simulink model "Simulink_EbolaControlSISO"  (R2021b)
settings: Solver=VariableStepAuto  StartTime=0.0  StopTime=1000.0  FixedStep=0.00126939799450362  RelTol=1e-3
model workspace (MAT data in the model file):
  Beta = 1.89e-07
  C = 8
  Delta = 0.0055
  P = 378
  U = 500
  Uu = 250
  V0 = 1.05
  u = 250
undefined symbols (not defined in the file or in its folder): sigbuilder_block
settings Model: Creator=Camilo  LastModifiedBy=Camilo
settings DataIOCC: SaveFormat=Array  OutputTimes=tout

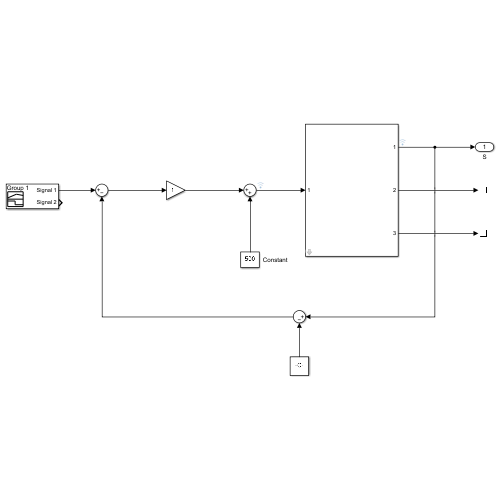
[thumbnail: Simulink's stored preview of the top-level diagram]
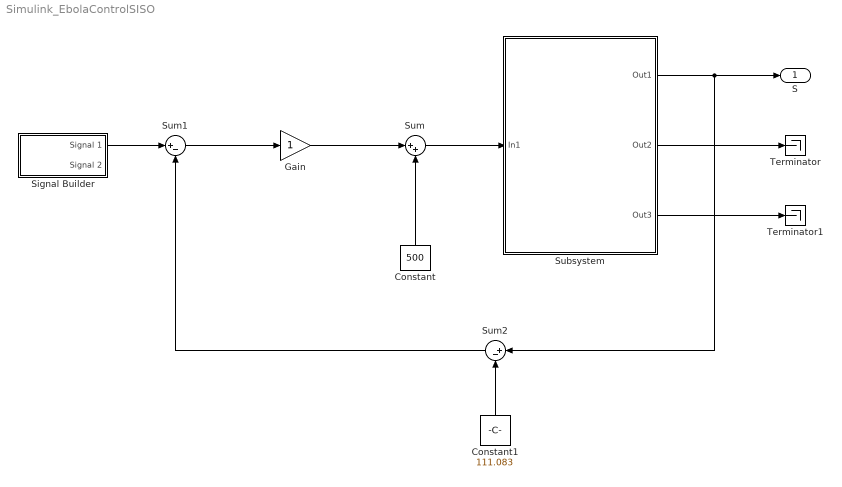
== system Simulink_EbolaControlSISO ==
  Constant : Constant  Value=500  VectorParams1D=off  SampleTime=-1
  Constant1 : Constant  Value=111.083
  Gain : Gain
  Signal Builder : Subsystem  Tag=STV Subsys  LoadFcn=sigbuilder_block('load',[429.6 149.4 550.8 400.2 ]);  StartFcn=sigbuilder_block('start');  StopFcn=sigbuilder_block('stop');  ClipboardFcn=sigbuilder_block('clipboard');  mask(Sigbuilder block){tuvar=[0:10]}
      mask help: Simulink:masks:SigbuilderBlock_MD
      mask init:
      | if ~strcmp(get_param(bdroot(gcbh),'SimulationStatus'),'stopped') tuvar = sigbuilder_block('maskInit'); end
      settings: CopyFcn=sigbuilder_block('copy');  DeleteFcn=sigbuilder_block('delete');  ModelCloseFcn=sigbuilder_block('modelClose');  PreSaveFcn=sigbuilder_block('preSave');  PauseFcn=sigbuilder_block('pause');  ContinueFcn=sigbuilder_block('continue');  NameChangeFcn=sigbuilder_block('namechange');  OpenFcn=sigbuilder_block('open',[429.6 149.4 550.8 400.2 ]);  CloseFcn=sigbuilder_block('close');
      mask Display: plot(0, 0, 100, 100,[2, 2, 32, 32, 2], [68, 8, 8, 68, 68],[32, 2], [38, 38], [32, 19, 2],[53, 60, 44], [32, 17, 17, 2],[16, 16, 31, 31]);txt = getActiveGroup(gcbh);text(2, 100, txt,'verticalAlignment', 'top');
  Subsystem : Subsystem  mask{V0=23560849.185935, Delta=1e-3, P=378, C=8.02, Beta=1.91e-7}
  Sum : Sum  Inputs=|++
  Sum1 : Sum  Inputs=|+-
  Sum2 : Sum  Inputs=|+-
  Terminator : Terminator
  Terminator1 : Terminator
  S : Outport
  wires:
  Subsystem/1(Out1) -> Sum2/1, S/1
  Subsystem/2(Out2) -> Terminator/1
  Subsystem/3(Out3) -> Terminator1/1
  Sum/1 -> Subsystem/1(In1)
  Constant/1 -> Sum/2
  Gain/1 -> Sum/1
  Sum1/1 -> Gain/1
  Constant1/1 -> Sum2/2
  Sum2/1 -> Sum1/2
  Signal Builder/1(Signal 1) -> Sum1/1

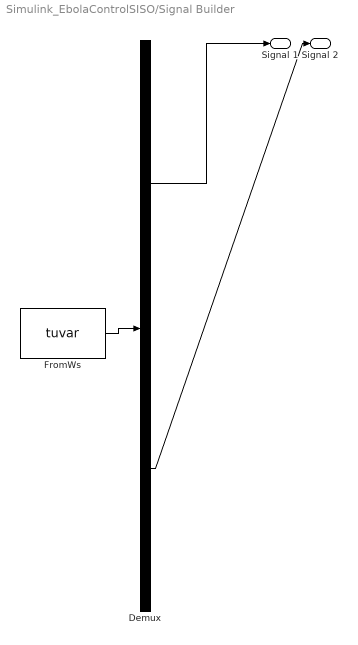
== system Simulink_EbolaControlSISO/Signal Builder ==
  Demux : Demux  Tag=STV Demux  Outputs=2
      settings: DisplayOption=none
  FromWs : FromWorkspace  Tag=STV FromWs  VariableName=tuvar
      SigBuilderData=|
      | common.afterFinalStr = 'Extrapolate'
      | common.sampleTime = 0
      | dataSet.timeRange = [0 10]
      | dataSet.name = 'Group 1'
      | sbobj.Groups.Name = 'Group 1'
      | sbobj.Groups.Signals(1).Name = 'Signal 1'
      | sbobj.Groups.Signals(1).XData = [0 10]
      | sbobj.Groups.Signals(1).YData = [0 0]
      | sbobj.Groups.Signals(2).Name = 'Signal 2'
      | sbobj.Groups.Signals(2).XData = [0 4 4 6 6 10]
      | sbobj.Groups.Signals(2).YData = [0 0 1 1 0 0]
  Signal 1 : Outport  Tag=STV Outport
  Signal 2 : Outport  Tag=STV Outport  Port=2
  wires:
  Demux/1 -> Signal 1/1
  FromWs/1 -> Demux/1
  Demux/2 -> Signal 2/1

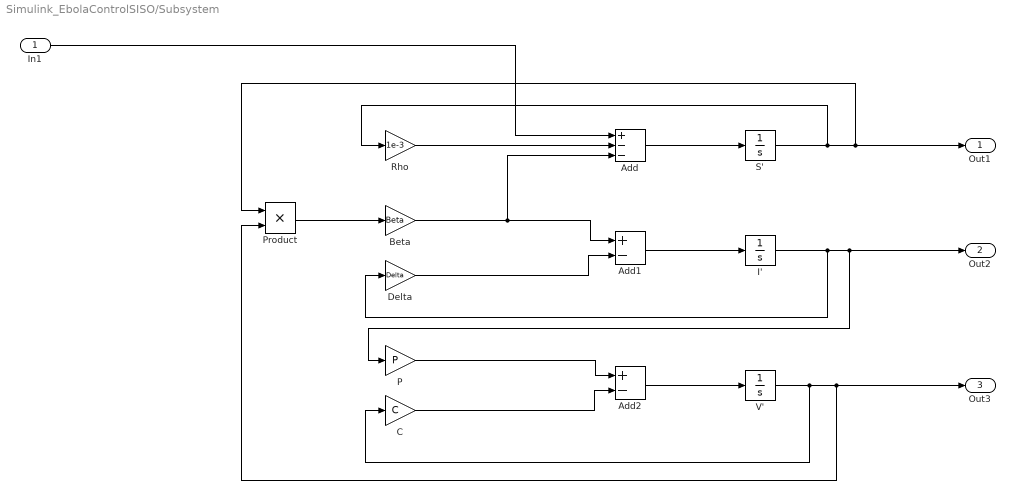
== system Simulink_EbolaControlSISO/Subsystem ==
  In1 : Inport
  Add : Sum  Inputs=+--
  Add1 : Sum  Inputs=+-
  Add2 : Sum  Inputs=+-
  Beta : Gain  Gain=Beta
  C : Gain  Gain=C
  Delta : Gain  Gain=Delta
  I' : Integrator  InitialCondition=4.99988917e+05  LimitOutput=on  LowerSaturationLimit=0
  P : Gain  Gain=P
  Product : Product
  Rho : Gain  Gain=1e-3
  S' : Integrator  InitialCondition=111.083  LimitOutput=on  LowerSaturationLimit=0
  V' : Integrator  InitialCondition=V0  LimitOutput=on  LowerSaturationLimit=0
  Out1 : Outport
  Out2 : Outport  Port=2
  Out3 : Outport  Port=3
  wires:
  Add/1 -> S'/1
  C/1 -> Add2/2
  Beta/1 -> Add1/1, Add/3
  I'/1 -> Out2/1, P/1, Delta/1
  P/1 -> Add2/1
  S'/1 -> Out1/1, Product/1, Rho/1
  Rho/1 -> Add/2
  V'/1 -> Out3/1, Product/2, C/1
  Add2/1 -> V'/1
  Product/1 -> Beta/1
  Add1/1 -> I'/1
  Delta/1 -> Add1/2
  In1/1 -> Add/1
